simulink model "mpm_blocks"  (R2023a)
settings: Solver=VariableStepAuto  StartTime=0.0  StopTime=10.0  RelTol=1e-3
undefined symbols (not defined in the file or in its folder): conv, es
(part 1 of 3)
settings Model: Creator=bartonsa  LastModifiedBy=smbar

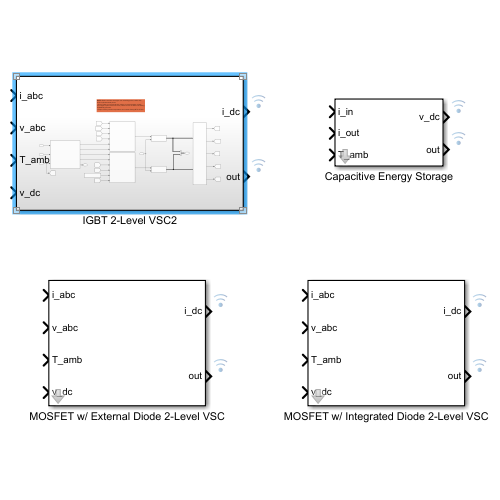
[thumbnail: Simulink's stored preview of the top-level diagram]
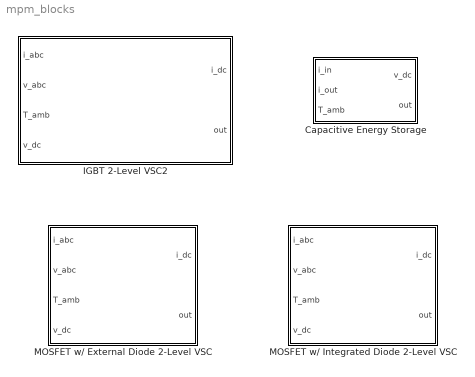
== system mpm_blocks ==
  Capacitive Energy Storage : Subsystem  mask{es=es(1)}
      mask prompts: es "Energy storage element number (i.e., es(n))"
      mask DialogControl DescGroupVar Prompt: Capacitive Energy Storage
      mask DialogControl DescTextVar Prompt: Models the thermal response of a capacitive energy storage element (i.e., supercapacitor, ultracapacitor, etc.).
  IGBT 2-Level VSC2 : Subsystem
  MOSFET w/ External Diode 2-Level VSC : Subsystem  mask{conv=conv(1)}
      mask prompts: conv "Converter name (i.e., conv(n))"
      mask DialogControl DescGroupVar Prompt: 2L VSC - MOSFET w/ ExternalDiode
      mask DialogControl DescTextVar Prompt: Models the thermal response of all switching devices in the power electronic converter.
      mask DialogControl DescTextVar2 Prompt: "out" is the junction temperature measurements for all converter devices.
      mask DialogControl DescTextVar3 Prompt: NOTE: i) Phase current is defined as flowing TOWARDS load ii) DC bus current is defined as flowing TOWARDS DC link iii) Assuming external anti-parallel diode, therefore no use of the body diode of the MOSFET.
  MOSFET w/ Integrated Diode 2-Level VSC : Subsystem  mask{conv=conv(1)}
      mask prompts: conv "Converter element (i.e., conv(n))"
      mask DialogControl DescGroupVar Prompt: 2L VSC - MOSFET w/ Integrated Diode
      mask DialogControl DescTextVar Prompt: Models the thermal response of all switching devices in the power electronic converter.
      mask DialogControl DescTextVar2 Prompt: "out" is the junction temperature measurements for all converter devices.
      mask DialogControl DescTextVar1 Prompt: NOTE: i) Phase current is defined as flowing TOWARDS load ii) DC bus current is defined as flowing TOWARDS DC link iii) Assuming no external anti-parallel diode, only the body diode of the MOSFET.

== system mpm_blocks/Capacitive Energy Storage ==
  note: Two-branch model of supercapacitor
      | Model derived from the work presented in Faranda et al., "A new parameter identification procedure for simplified double layer capacitor two-branch model," 2010
  i_in : Inport
  i_out : Inport  Port=2
  T_amb : Inport  Port=3
  Bus Creator : BusCreator  Inputs=1
  Constant : Constant  Value=es.c_0
  Constant5 : Constant  Value=es.k_v
  Constant6 : Constant  Value=es.c_2
  Divide : Product  Inputs=*/
  Divide1 : Product  Inputs=*/
  Gain : Gain  Gain=1/es.r_0
  Gain1 : Gain  Gain=1/es.r_2
  Gain2 : Gain  Gain=1/es.r_0
  Gain3 : Gain  Gain=1/es.r_2
  Gain4 : Gain  Gain=1/((1/es.r_0)+(1/es.r_2))
  Gain5 : Gain  Gain=1/es.n_p
  Gain6 : Gain  Gain=es.n_s
  Gain7 : Gain  Gain=es.r_0
  Gain8 : Gain  Gain=es.r_2
  Gain9 : Gain  Gain=es.theta
  Integrator : Integrator  InitialCondition=es.v_0
  Integrator1 : Integrator  InitialCondition=es.v_0
  Product : Product
  Square : Math  Operator=square
  Square1 : Math  Operator=square
  Sum : Sum
  Sum1 : Sum
  Sum2 : Sum  Inputs=+-
  Sum3 : Sum  Inputs=+-
  Sum4 : Sum  Inputs=+++
  Sum5 : Sum  Inputs=|++
  Sum6 : Sum
  v_dc : Outport
  out : Outport  Port=2
  wires:
  Bus Creator/1 -> out/1
  Sum5/1 -> Bus Creator/1  "T"
  T_amb/1 -> Sum5/2
  Gain9/1 -> Sum5/1
  Sum6/1 -> Gain9/1  "P_loss"
  Gain7/1 -> Sum6/1
  Gain8/1 -> Sum6/2
  [i_2] -> Square1/1
  Square1/1 -> Gain8/1
  Square/1 -> Gain7/1
  [i_1] -> Square/1
  Gain6/1 -> v_dc/1  "v_dc"
  Gain5/1 -> Sum4/1  "i_cell"
  Sum4/1 -> Gain4/1
  Gain3/1 -> Sum4/2
  Gain2/1 -> Sum4/3
  Integrator1/1 -> Gain3/1, Sum3/2  "v_2"
  Constant6/1 -> Divide1/2
  Divide1/1 -> Integrator1/1  "d_v2"
  Gain1/1 -> [i_2], Divide1/1  "i_2"
  Sum3/1 -> Gain1/1
  Integrator/1 -> Product/1, Sum2/2, Gain2/1  "v_1"
  Divide/1 -> Integrator/1  "d_v1"
  Gain/1 -> Divide/1, [i_1]  "i_1"
  Sum2/1 -> Gain/1
  Gain4/1 -> Sum3/1, Sum2/1, Gain6/1  "v_cell"
  Sum1/1 -> Divide/2
  Product/1 -> Sum1/2
  Constant5/1 -> Product/2
  Constant/1 -> Sum1/1
  i_in/1 -> Sum/1
  Sum/1 -> Gain5/1  "i_c"
  i_out/1 -> Sum/2

== system mpm_blocks/IGBT 2-Level VSC2 ==
  note: NOTE: Model considers averages over switching period, rather than electrical fundamental period.
      | - Inputs: Phase current and phase voltage (or desired phase voltage from output of pwm reference block). Phase current is defined as flowing TOWARDS generator.
      | - Output: Device junction temperature and current flowing INTO DC link.
  i_abc : Inport
  v_abc : Inport  Port=2
  T_amb : Inport  Port=3
  v_dc : Inport  Port=4
  Bus Creator : BusCreator  Inputs=2
  Constant5 : Constant  Value=conv.dev(2).Q_rr*conv.v_dc
  DIODE Loss Modeling : Subsystem
  Duty & Current Calculation : Subsystem
  IGBT Loss Modeling : Subsystem
  Thermal Impacts : Subsystem
  Thermal Model : Subsystem  mask{dev=conv.dev(1)}
      mask prompts: dev "Device number (i.e., dev(n))"
      mask DialogControl DescGroupVar Prompt: Device Thermal Model
      mask DialogControl DescTextVar Prompt: Thermal model of the specific device (assuming no thermal dependence between the switching device and diode). Note that dev(1) is typically the switch (e.g., MOSFET or IGBT) and dev(2) is the diode.
  Thermal Model1 : Subsystem  mask{dev=conv.dev(1)}
      mask prompts: dev "Device number (i.e., dev(n))"
      mask DialogControl DescGroupVar Prompt: Device Thermal Model
      mask DialogControl DescTextVar Prompt: Thermal model of the specific device (assuming no thermal dependence between the switching device and diode). Note that dev(1) is typically the switch (e.g., MOSFET or IGBT) and dev(2) is the diode.
  i_dc : Outport
  out : Outport  Port=2
  wires:
  Thermal Impacts/3(v_ce) -> [v_ce0]  "v_ce0"
  Thermal Impacts/4(r_dio) -> [r_dio]  "r_dio"
  Thermal Impacts/2(E_Qsw) -> [E_Qsw]  "E_Qsw"
  Thermal Model/1(T_j) -> Thermal Impacts/1(T_Q), Bus Creator/1  "T_Q"
  T_amb/1 -> Thermal Model/2(T_amb), Thermal Model1/2(T_amb)
  IGBT Loss Modeling/1(P_Q) -> Thermal Model/1(P_loss)  "P_M"
  Thermal Impacts/1(r_on) -> [r_on]  "r_on"
  Thermal Model1/1(T_j) -> Thermal Impacts/2(T_D), Bus Creator/2  "T_D"
  Thermal Impacts/5(v_th) -> [v_th]  "v_th"
  Bus Creator/1 -> out/1
  DIODE Loss Modeling/1(P_D) -> Thermal Model1/1(P_loss)  "P_D"
  [v_ce0] -> IGBT Loss Modeling/4(v_ce0)  "r_ds"
  [r_on] -> IGBT Loss Modeling/3(r_on)  "r_ds"
  [E_Qsw] -> IGBT Loss Modeling/2(E_sw)  "E_sw"
  [v_dc] -> IGBT Loss Modeling/1(v_dc)
  [v_dc] -> DIODE Loss Modeling/6(v_dc)  "v_dc"
  [v_th] -> DIODE Loss Modeling/4(v_th)  "v_th"
  [r_dio] -> DIODE Loss Modeling/3(r_dio)  "r_dio"
  Constant5/1 -> DIODE Loss Modeling/5(E_rr)  "E_rr"
  Duty & Current Calculation/4(i_D) -> DIODE Loss Modeling/2(i_D)  "i_D"
  Duty & Current Calculation/3(d_D) -> DIODE Loss Modeling/1(d_D)  "d_D"
  Duty & Current Calculation/2(i_Q) -> IGBT Loss Modeling/6(i_Q)  "i_Q"
  Duty & Current Calculation/1(d_Q) -> IGBT Loss Modeling/5(d_Q)  "d_Q"
  v_dc/1 -> Duty & Current Calculation/3(v_dc), [v_dc]
  i_abc/1 -> Duty & Current Calculation/1(i_s)
  v_abc/1 -> Duty & Current Calculation/2(v_s)
  Duty & Current Calculation/5(i_dc) -> i_dc/1

== system mpm_blocks/MOSFET w// External Diode 2-Level VSC ==
  note: NOTE: Model considers averages over switching period, rather than electrical fundamental period.
      | - Inputs: Phase current and phase voltage (or desired phase voltage from output of pwm reference block). Phase current is defined as flowing TOWARDS generator.
      | - Output: Device junction temperature and current flowing INTO DC link.
  i_abc : Inport
  v_abc : Inport  Port=2
  T_amb : Inport  Port=3
  v_dc : Inport  Port=4
  Bus Creator : BusCreator  Inputs=2
  Calculate Duty & Currents : Subsystem
      settings: PortSchema="{\"entries\":[{\"content\":{\"sides\":[{\"content\":{\"connectorIds\":[\"In1\",\"In2\",\"In3\"]},\"type\":\"ConnectorPlacement.EquallySpacedRectSide\",\"uuid\":\"d0795c63-5d1f-4e94-8f4f-403311821ded\"},{\"content\":{\"connectorIds\":[\"Out1\",\"Out2\",\"Out3\",\"Out4\",\"Out5\"],\"side\":\"RIGHT\"},\"type\":\"ConnectorPlacement.EquallySpacedRectSide\",\"uuid\":\"545dd18c-9caf-4cea-89fb-dae66879e352\"},{\"content\":{\"connectorIds\":[\"In4\",\"In5\",\"In6\"],\"side\":\"TOP\"},\"type\":\"ConnectorPlacement.EquallySpacedRectSide\",\"uuid\":\"9e7296e6-8783-47bd-a40b-6e0da827b704\"}]},\"type\":\"ConnectorPlacement.EquallySpacedConnector\",\"uuid\":\"8ebf9a6f-bb7f-485d-8612-a50ce46f0952\"}],\"packageUris\":[\"http://schema.mathworks.com/mf0/Connector/R2020b\"],\"version\":\"1.0\"}"
  Constant5 : Constant  Value=conv.dev(2).Q_rr*conv.v_dc
  DIODE Loss Modeling : Subsystem
  MOSFET Loss Modeling : Subsystem
  Thermal Impacts : Subsystem
  Thermal Model : Subsystem  mask{dev=conv.dev(1)}
      mask prompts: dev "Device number (i.e., dev(n))"
      mask DialogControl DescGroupVar Prompt: Device Thermal Model
      mask DialogControl DescTextVar Prompt: Thermal model of the specific device (assuming no thermal dependence between MOSFET and diode). Note that dev(1) is typically the switch (e.g., MOSFET or IGBT) and dev(2) is the diode.
  Thermal Model 1 : Subsystem  mask{dev=conv.dev(2)}
      mask prompts: dev "Device number (i.e., dev(n))"
      mask DialogControl DescGroupVar Prompt: Device Thermal Model
      mask DialogControl DescTextVar Prompt: Thermal model of the specific device (assuming no thermal dependence between MOSFET and diode). Note that dev(1) is typically the switch (e.g., MOSFET or IGBT) and dev(2) is the diode.
  i_dc : Outport
  out : Outport  Port=2
  wires:
  [r_ds] -> MOSFET Loss Modeling/3(r_ds)  "r_ds"
  DIODE Loss Modeling/1(P_D) -> Thermal Model 1/1(P_loss)  "P_D"
  T_amb/1 -> Thermal Model/2(T_amb), Thermal Model 1/2(T_amb)
  Thermal Impacts/4(v_th) -> [v_th]  "v_th"
  MOSFET Loss Modeling/1(P_M) -> Thermal Model/1(P_loss)  "P_M"
  Thermal Model/1(T_j) -> Bus Creator/1, Thermal Impacts/1(T_m)  "T_m"
  Thermal Impacts/3(r_dio) -> [r_dio]  "r_dio"
  Thermal Impacts/2(E_Qsw) -> [E_Qsw]  "E_Qsw"
  Constant5/1 -> DIODE Loss Modeling/5(E_rr)  "E_rr"
  [E_Qsw] -> MOSFET Loss Modeling/2(E_sw)  "E_sw"
  [v_th] -> DIODE Loss Modeling/4(v_th)  "v_th"
  [r_dio] -> DIODE Loss Modeling/3(r_dio)  "r_dio"
  Thermal Impacts/1(r_dson) -> [r_ds]  "r_dson"
  Calculate Duty & Currents/4(i_D) -> DIODE Loss Modeling/2(i_D)  "i_D"
  Calculate Duty & Currents/2(i_M) -> MOSFET Loss Modeling/5(i_M)  "i_M"
  Calculate Duty & Currents/1(d_M) -> MOSFET Loss Modeling/4(d_M)  "d_M"
  [r_ds] -> Calculate Duty & Currents/1(r_ds)  "r_ds"
  [v_th] -> Calculate Duty & Currents/2(v_th)  "v_th"
  [r_dio] -> Calculate Duty & Currents/3(r_dio)  "r_dio"
  Calculate Duty & Currents/3(d_D) -> DIODE Loss Modeling/1(d_D)  "d_D"
  Thermal Model 1/1(T_j) -> Thermal Impacts/2(T_d), Bus Creator/2  "T_d"
  Bus Creator/1 -> out/1
  v_dc/1 -> [v_dc], Calculate Duty & Currents/6(v_dc)
  i_abc/1 -> Calculate Duty & Currents/5(i_s)
  v_abc/1 -> Calculate Duty & Currents/4(v_s)
  Calculate Duty & Currents/5(i_dc) -> i_dc/1
  [v_dc] -> DIODE Loss Modeling/6(v_dc)  "v_dc"
  [v_dc] -> MOSFET Loss Modeling/1(v_dc)

== system mpm_blocks/MOSFET w// Integrated Diode 2-Level VSC ==
  note: NOTE: Model considers averages over switching period, rather than electrical fundamental period.
      | - Inputs: Phase current and phase voltage (or desired phase voltage from output of pwm reference block). Phase current is defined as flowing TOWARDS generator.
      | - Output: Device junction temperature and current flowing INTO DC link.
  i_abc : Inport
  v_abc : Inport  Port=2
  T_amb : Inport  Port=3
  v_dc : Inport  Port=4
  Calculate Duty & Currents : Subsystem
      settings: PortSchema="{\"entries\":[{\"content\":{\"sides\":[{\"content\":{\"connectorIds\":[\"In1\",\"In2\",\"In3\"]},\"type\":\"ConnectorPlacement.EquallySpacedRectSide\",\"uuid\":\"d0795c63-5d1f-4e94-8f4f-403311821ded\"},{\"content\":{\"connectorIds\":[\"Out1\",\"Out2\",\"Out3\",\"Out4\",\"Out5\"],\"side\":\"RIGHT\"},\"type\":\"ConnectorPlacement.EquallySpacedRectSide\",\"uuid\":\"545dd18c-9caf-4cea-89fb-dae66879e352\"},{\"content\":{\"connectorIds\":[\"In4\",\"In5\",\"In6\"],\"side\":\"TOP\"},\"type\":\"ConnectorPlacement.EquallySpacedRectSide\",\"uuid\":\"9e7296e6-8783-47bd-a40b-6e0da827b704\"}]},\"type\":\"ConnectorPlacement.EquallySpacedConnector\",\"uuid\":\"8ebf9a6f-bb7f-485d-8612-a50ce46f0952\"}],\"packageUris\":[\"http://schema.mathworks.com/mf0/Connector/R2020b\"],\"version\":\"1.0\"}"
  Constant5 : Constant  Value=conv.dev(2).Q_rr*conv.v_dc
  DE Loss Modeling : Subsystem
      settings: PortSchema="{\"entries\":[{\"content\":{\"sides\":[{\"content\":{\"connectorIds\":[\"In1\",\"In2\"]},\"type\":\"ConnectorPlacement.EquallySpacedRectSide\",\"uuid\":\"33e83bff-44ec-4dc6-9bbd-b270e5176242\"},{\"content\":{\"connectorIds\":[\"Out1\"],\"side\":\"RIGHT\"},\"type\":\"ConnectorPlacement.EquallySpacedRectSide\",\"uuid\":\"aed5fe4c-6bb6-427c-a555-2403a405bda4\"},{\"content\":{\"side\":\"TOP\"},\"type\":\"ConnectorPlacement.EquallySpacedRectSide\",\"uuid\":\"31452d4f-f1d8-4db9-9193-98611747bca7\"},{\"content\":{\"connectorIds\":[\"In3\",\"In4\",\"In5\",\"In6\"],\"side\":\"BOTTOM\"},\"type\":\"ConnectorPlacement.EquallySpacedRectSide\",\"uuid\":\"6203e927-6eb2-4c43-a609-9ad9799e7e1f\"}]},\"type\":\"ConnectorPlacement.EquallySpacedConnector\",\"uuid\":\"1e03b39d-f61e-43a7-b650-f6897d256e67\"}],\"packageUris\":[\"http://schema.mathworks.com/mf0/Connector/R2020b\"],\"version\":\"1.0\"}"
  MOSFET Loss Modeling : Subsystem
      settings: PortSchema="{\"entries\":[{\"content\":{\"sides\":[{\"content\":{\"connectorIds\":[\"In1\",\"In2\"]},\"type\":\"ConnectorPlacement.EquallySpacedRectSide\",\"uuid\":\"be72776b-5d84-4e7d-87ca-7034f165601e\"},{\"content\":{\"connectorIds\":[\"Out1\"],\"side\":\"RIGHT\"},\"type\":\"ConnectorPlacement.EquallySpacedRectSide\",\"uuid\":\"5d971d04-5834-4819-98b1-31b200ab7220\"},{\"content\":{\"connectorIds\":[\"In3\",\"In4\",\"In5\"],\"side\":\"TOP\"},\"type\":\"ConnectorPlacement.EquallySpacedRectSide\",\"uuid\":\"65eaa64d-9a38-435b-9775-bcfd5a35040a\"}]},\"type\":\"ConnectorPlacement.EquallySpacedConnector\",\"uuid\":\"b4736152-0e1c-4fdb-a43a-e03615dd6111\"}],\"packageUris\":[\"http://schema.mathworks.com/mf0/Connector/R2020b\"],\"version\":\"1.0\"}"
  Sum1 : Sum
  Thermal Impacts : Subsystem
  Thermal Model : Subsystem
  i_dc : Outport
  out : Outport  Port=2
  wires:
  MOSFET Loss Modeling/1(P_M) -> Sum1/1  "P_M"
  [r_ds] -> MOSFET Loss Modeling/3(r_ds)  "r_ds"
  DE Loss Modeling/1(P_D) -> Sum1/2  "P_D"
  T_amb/1 -> Thermal Model/2(T_amb)
  Thermal Impacts/4(v_th) -> [v_th]  "v_th"
  Sum1/1 -> Thermal Model/1(P_loss)  "P_dev"
  Thermal Model/1(T_j) -> out/1, Thermal Impacts/1(T_j)  "T_j"
  Thermal Impacts/3(r_dio) -> [r_dio]  "r_dio"
  Thermal Impacts/2(E_Qsw) -> [E_Qsw]  "E_Qsw"
  Constant5/1 -> DE Loss Modeling/6(E_rr)  "E_rr"
  [E_Qsw] -> MOSFET Loss Modeling/4(E_sw)  "E_sw"
  [v_th] -> DE Loss Modeling/4(v_th)  "v_th"
  i_abc/1 -> Calculate Duty & Currents/5(i_s)
  [r_dio] -> DE Loss Modeling/3(r_dio)  "r_dio"
  Thermal Impacts/1(r_dson) -> [r_ds]  "r_dson"
  Calculate Duty & Currents/4(i_D) -> DE Loss Modeling/2(i_D)  "i_D"
  Calculate Duty & Currents/2(i_M) -> MOSFET Loss Modeling/2(i_M)  "i_M"
  Calculate Duty & Currents/1(d_M) -> MOSFET Loss Modeling/1(d_M)  "d_M"
  v_abc/1 -> Calculate Duty & Currents/4(v_s)
  [r_ds] -> Calculate Duty & Currents/1(r_ds)  "r_ds"
  [v_th] -> Calculate Duty & Currents/2(v_th)  "v_th"
  [r_dio] -> Calculate Duty & Currents/3(r_dio)  "r_dio"
  Calculate Duty & Currents/3(d_D) -> DE Loss Modeling/1(d_D)  "d_D"
  v_dc/1 -> [v_dc], Calculate Duty & Currents/6(v_dc)
  Calculate Duty & Currents/5(i_dc) -> i_dc/1
  [v_dc] -> MOSFET Loss Modeling/5(v_dc)  "v_dc"
  [v_dc] -> DE Loss Modeling/5(v_dc)  "v_dc"

== system mpm_blocks/IGBT 2-Level VSC2/DIODE Loss Modeling ==
  d_D : Inport
  i_D : Inport  Port=2
  r_dio : Inport  Port=3
  v_th : Inport  Port=4
  E_rr : Inport  Port=5
  v_dc : Inport  Port=6
  Gain : Gain  Gain=1/conv.dev(2).V_ref
  Gain3 : Gain  Gain=1/conv.dev(2).I_ref
  Gain4 : Gain  Gain=conv.f_sw
  Product : Product
  Product3 : Product  Inputs=3
  Product6 : Product  Inputs=3
  Product8 : Product
  Sqrt : Sqrt
  Square2 : Math  Operator=square
  Sum : Sum
  Sum2 : Sum
  P_D : Outport
  wires:
  v_dc/1 -> Gain/1
  Product/1 -> Gain3/1, Product8/1  "i_D_avg"
  i_D/1 -> Square2/1, Product/2  "i_D"
  d_D/1 -> Product6/2, Product/1  "d_D"
  Sqrt/1 -> Product3/3  "iscale"
  Gain3/1 -> Sqrt/1
  Gain/1 -> Product3/2  "vscale"
  Product6/1 -> Sum/1
  Product8/1 -> Sum/2
  Square2/1 -> Product6/3
  Sum/1 -> Sum2/1  "P_CD"
  Gain4/1 -> Sum2/2  "P_SD"
  r_dio/1 -> Product6/1
  Product3/1 -> Gain4/1
  Sum2/1 -> P_D/1  "P_D"
  v_th/1 -> Product8/2
  E_rr/1 -> Product3/1

== system mpm_blocks/IGBT 2-Level VSC2/Duty & Current Calculation ==
  note: Duty Cycle Estimation
  i_s : Inport
  v_s : Inport  Port=2
  v_dc : Inport  Port=3
  Calculate Device Currents : MATLAB Function  TreatAsAtomicUnit=on
  Constant : Constant
  Constant2 : Constant
  Constant3 : Constant  Value=2*conv.t_d*conv.f_sw
  Constant4 : Constant  Value=2*conv.t_d*conv.f_sw
  Divide : Product  Inputs=*/
  Gain : Gain  Gain=-1
  Gain1 : Gain  Gain=1/2
  Gain2 : Gain  Gain=2
  MATLAB Function3 : MATLAB Function  TreatAsAtomicUnit=on
  Mux : Mux  Inputs=2
  Product : Product
  Product1 : Product
  Selector : Selector  InputPortWidth=6  IndexOptions=Index vector (dialog)  Indices=[1 2 3]  OutputSizes=1
  Selector1 : Selector  InputPortWidth=6  IndexOptions=Index vector (dialog)  Indices=[1 2 3]  OutputSizes=1
  Subtract : Sum  Inputs=+-
  Subtract1 : Sum  Inputs=-+-
  Sum of Elements : Sum  Inputs=+
  Sum1 : Sum  Inputs=+-+
  d_Q : Outport
  i_Q : Outport  Port=2
  d_D : Outport  Port=3
  i_D : Outport  Port=4
  i_dc : Outport  Port=5
  wires:
  Calculate Device Currents/4(d_D) -> d_D/1, Product1/2  "d_D"
  Calculate Device Currents/3(i_D) -> Product1/1, i_D/1  "i_D"
  Calculate Device Currents/1(i_Q) -> Product/1, i_Q/1  "i_Q"
  Selector1/1 -> Subtract/2
  Selector/1 -> Subtract/1
  Subtract/1 -> Sum of Elements/1  "diff"
  Sum of Elements/1 -> Gain/1
  Gain/1 -> i_dc/1  "i_dc"
  Product/1 -> Selector/1  "iQ_avg"
  Product1/1 -> Selector1/1  "iD_avg"
  i_s/1 -> Calculate Device Currents/3(i_s)
  Mux/1 -> Calculate Device Currents/1(d_Q)  "d_Q"
  Calculate Device Currents/2(d_Qnew) -> d_Q/1, Product/2  "d_Q"
  MATLAB Function3/1(y) -> Sum1/3
  Constant/1 -> Sum1/1
  v_s/1 -> Gain2/1  "v_s"
  Constant2/1 -> Subtract1/2
  Gain1/1 -> Mux/1, Subtract1/1  "d_H"
  Divide/1 -> MATLAB Function3/1(u)  "m_a"
  Sum1/1 -> Gain1/1
  Constant4/1 -> Calculate Device Currents/2(d_deadTime), Subtract1/3  "d_deadTime"
  Subtract1/1 -> Mux/2  "d_L"
  Constant3/1 -> Sum1/2
  Gain2/1 -> Divide/1
  v_dc/1 -> Divide/2

== system mpm_blocks/IGBT 2-Level VSC2/IGBT Loss Modeling ==
  note: P_cond = v_ce*I_avg + r_on*I_rms^2
  v_dc : Inport
  E_sw : Inport  Port=2
  r_on : Inport  Port=3
  v_ce0 : Inport  Port=4
  d_Q : Inport  Port=5
  i_Q : Inport  Port=6
  Abs : Abs  SaturateOnIntegerOverflow=off
  Constant : Constant  Value=conv.dev(1).k_v
  Gain : Gain  Gain=1/conv.dev(1).V_ref
  Gain1 : Gain  Gain=conv.f_sw
  Gain2 : Gain  Gain=1/conv.dev(1).I_ref
  Power : Math  Operator=pow
  Product : Product
  Product1 : Product
  Product10 : Product  Inputs=3
  Product2 : Product
  Product4 : Product  Inputs=3
  Square : Math  Operator=square
  Sum : Sum
  Sum1 : Sum
  P_Q : Outport
  wires:
  Product1/1 -> Sum/1
  Product4/1 -> Sum/2  "P_CQ"
  Product2/1 -> Product1/2  "i_Qavg"
  v_ce0/1 -> Product1/1
  v_dc/1 -> Gain/1
  Gain/1 -> Power/1
  Constant/1 -> Power/2
  Product/1 -> Abs/1  "i_Qavg"
  d_Q/1 -> Product2/1, Product4/2, Product/2  "d"
  Abs/1 -> Gain2/1
  Sum1/1 -> P_Q/1  "P_Q"
  E_sw/1 -> Product10/1
  i_Q/1 -> Product/1, Square/1, Product2/2  "i_Q"
  Gain1/1 -> Sum1/2  "P_SQ"
  r_on/1 -> Product4/1
  Power/1 -> Product10/3  "vscale"
  Product10/1 -> Gain1/1
  Square/1 -> Product4/3
  Gain2/1 -> Product10/2  "iscale"
  Sum/1 -> Sum1/1  "P_CQ"

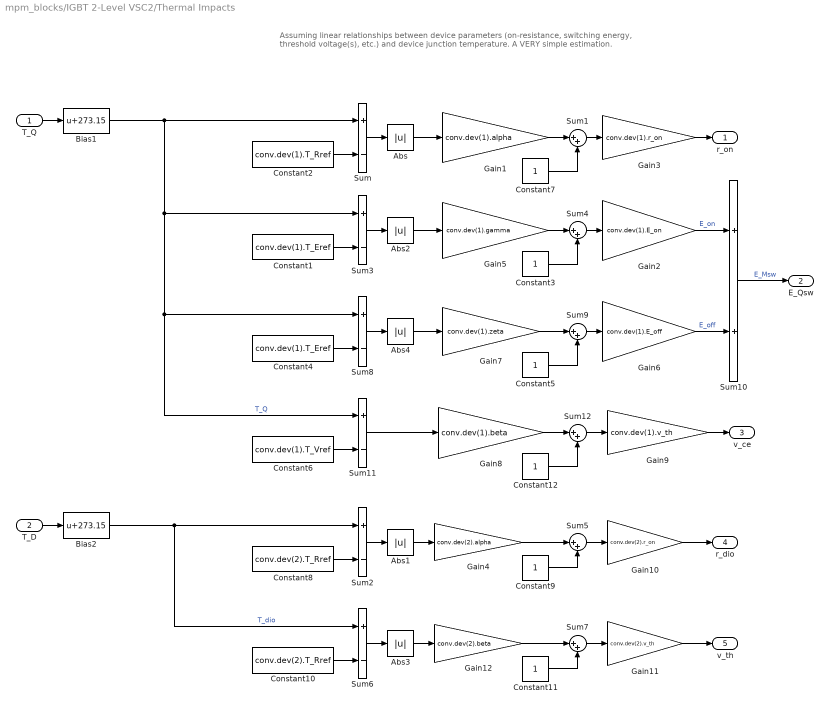
== system mpm_blocks/IGBT 2-Level VSC2/Thermal Impacts ==
  note: Assuming linear relationships between device parameters (on-resistance, switching energy, threshold voltage(s), etc.) and device junction temperature. A VERY simple estimation.
  T_Q : Inport
  T_D : Inport  Port=2
  Abs{,1..4} (5 alike) : Abs  SaturateOnIntegerOverflow=off
  Bias1 : Bias  Bias=273.15  SaturateOnIntegerOverflow=off
  Bias2 : Bias  Bias=273.15  SaturateOnIntegerOverflow=off
  Constant1 : Constant  Value=conv.dev(1).T_Eref
  Constant10 : Constant  Value=conv.dev(2).T_Rref
  Constant{3,5,7,9,11..12} (6 alike) : Constant
  Constant2 : Constant  Value=conv.dev(1).T_Rref
  Constant4 : Constant  Value=conv.dev(1).T_Eref
  Constant6 : Constant  Value=conv.dev(1).T_Vref
  Constant8 : Constant  Value=conv.dev(2).T_Rref
  Gain1 : Gain  Gain=conv.dev(1).alpha
  Gain10 : Gain  Gain=conv.dev(2).r_on
  Gain11 : Gain  Gain=conv.dev(2).v_th
  Gain12 : Gain  Gain=conv.dev(2).beta
  Gain2 : Gain  Gain=conv.dev(1).E_on
  Gain3 : Gain  Gain=conv.dev(1).r_on
  Gain4 : Gain  Gain=conv.dev(2).alpha
  Gain5 : Gain  Gain=conv.dev(1).gamma
  Gain6 : Gain  Gain=conv.dev(1).E_off
  Gain7 : Gain  Gain=conv.dev(1).zeta
  Gain8 : Gain  Gain=conv.dev(1).beta
  Gain9 : Gain  Gain=conv.dev(1).v_th
  Sum{,2..3,6,8,11} (6 alike) : Sum  Inputs=+-
  Sum{1,4..5,7,9,12} (6 alike) : Sum  Inputs=|++
  Sum10 : Sum
  r_on : Outport
  E_Qsw : Outport  Port=2
  v_ce : Outport  Port=3
  r_dio : Outport  Port=4
  v_th : Outport  Port=5
  wires:
  Sum11/1 -> Gain8/1
  Constant12/1 -> Sum12/2
  Sum12/1 -> Gain9/1
  Gain9/1 -> v_ce/1
  Gain8/1 -> Sum12/1
  Constant6/1 -> Sum11/2
  T_D/1 -> Bias2/1
  Bias2/1 -> Sum2/1, Sum6/1  "T_dio"
  T_Q/1 -> Bias1/1
  Bias1/1 -> Sum/1, Sum3/1, Sum8/1, Sum11/1  "T_Q"
  Sum10/1 -> E_Qsw/1  "E_Msw"
  Gain7/1 -> Sum9/1
  Sum8/1 -> Abs4/1
  Constant5/1 -> Sum9/2
  Sum9/1 -> Gain6/1
  Gain6/1 -> Sum10/2  "E_off"
  Abs4/1 -> Gain7/1
  Constant4/1 -> Sum8/2
  Constant1/1 -> Sum3/2
  Sum4/1 -> Gain2/1
  Gain2/1 -> Sum10/1  "E_on"
  Abs2/1 -> Gain5/1
  Gain5/1 -> Sum4/1
  Constant3/1 -> Sum4/2
  Sum3/1 -> Abs2/1
  Abs3/1 -> Gain12/1
  Constant2/1 -> Sum/2
  Constant11/1 -> Sum7/2
  Gain11/1 -> v_th/1
  Sum7/1 -> Gain11/1
  Constant10/1 -> Sum6/2
  Gain12/1 -> Sum7/1
  Sum6/1 -> Abs3/1
  Abs/1 -> Gain1/1
  Gain1/1 -> Sum1/1
  Sum1/1 -> Gain3/1
  Constant7/1 -> Sum1/2
  Sum2/1 -> Abs1/1
  Constant8/1 -> Sum2/2
  Constant9/1 -> Sum5/2
  Gain4/1 -> Sum5/1
  Abs1/1 -> Gain4/1
  Sum5/1 -> Gain10/1
  Gain10/1 -> r_dio/1
  Gain3/1 -> r_on/1
  Sum/1 -> Abs/1

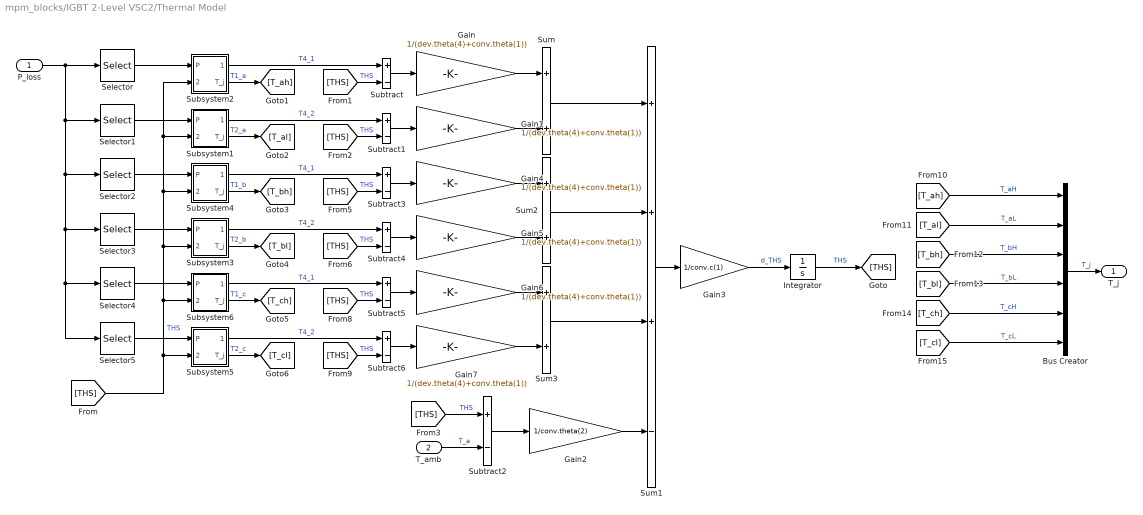
== system mpm_blocks/IGBT 2-Level VSC2/Thermal Model ==
  P_loss : Inport
  T_amb : Inport  Port=2
  Bus Creator : BusCreator  Inputs=6
  Gain{,1,4..7} (6 alike) : Gain  Gain=1/(dev.theta(4)+conv.theta(1))
  Gain2 : Gain  Gain=1/conv.theta(2)
  Gain3 : Gain  Gain=1/conv.c(1)
  Integrator : Integrator  InitialCondition=conv.T_init-273.15
  Selector : Selector  InputPortWidth=6  IndexOptions=Index vector (dialog)  Indices=1  OutputSizes=1
  Selector1 : Selector  InputPortWidth=6  IndexOptions=Index vector (dialog)  Indices=4  OutputSizes=1
  Selector2 : Selector  InputPortWidth=6  IndexOptions=Index vector (dialog)  Indices=2  OutputSizes=1
  Selector3 : Selector  InputPortWidth=6  IndexOptions=Index vector (dialog)  Indices=5  OutputSizes=1
  Selector4 : Selector  InputPortWidth=6  IndexOptions=Index vector (dialog)  Indices=3  OutputSizes=1
  Selector5 : Selector  InputPortWidth=6  IndexOptions=Index vector (dialog)  Indices=6  OutputSizes=1
  Subsystem1 : Subsystem
  Subsystem2 : Subsystem
  Subsystem3 : Subsystem
  Subsystem4 : Subsystem
  Subsystem5 : Subsystem
  Subsystem6 : Subsystem
  Subtract{,1..6} (7 alike) : Sum  Inputs=+-
  Sum : Sum
  Sum1 : Sum  Inputs=+++-
  Sum2 : Sum
  Sum3 : Sum
  T_j : Outport
  wires:
  [THS] -> Subsystem5/2(THS), Subsystem6/2(THS), Subsystem3/2(THS), Subsystem4/2(THS), Subsystem1/2(THS), Subsystem2/2(THS)  "THS"
  Selector2/1 -> Subsystem4/1(P)
  Selector1/1 -> Subsystem1/1(P)
  Selector5/1 -> Subsystem5/1(P)
  Selector4/1 -> Subsystem6/1(P)
  Selector3/1 -> Subsystem3/1(P)
  Selector/1 -> Subsystem2/1(P)
  [T_bh] -> Bus Creator/3  "T_bH"
  Bus Creator/1 -> T_j/1  "T_j"
  [T_cl] -> Bus Creator/6  "T_cL"
  [T_al] -> Bus Creator/2  "T_aL"
  [T_bl] -> Bus Creator/4  "T_bL"
  [T_ch] -> Bus Creator/5  "T_cH"
  [T_ah] -> Bus Creator/1  "T_aH"
  P_loss/1 -> Selector/1, Selector1/1, Selector2/1, Selector3/1, Selector4/1, Selector5/1
  Subsystem6/2(T_j) -> [T_ch]  "T1_c"
  Subtract1/1 -> Gain1/1
  Subtract3/1 -> Gain4/1
  Gain3/1 -> Integrator/1  "d_THS"
  Sum2/1 -> Sum1/2
  Subsystem4/1(T_c) -> Subtract3/1  "T4_1"
  Subsystem3/1(T_c) -> Subtract4/1  "T4_2"
  Sum3/1 -> Sum1/3
  Subsystem4/2(T_j) -> [T_bh]  "T1_b"
  Gain1/1 -> Sum/2
  Gain5/1 -> Sum2/2
  [THS] -> Subtract/2  "THS"
  Subtract2/1 -> Gain2/1
  [THS] -> Subtract3/2  "THS"
  Subtract5/1 -> Gain6/1
  [THS] -> Subtract4/2  "THS"
  Subsystem5/1(T_c) -> Subtract6/1  "T4_2"
  Gain4/1 -> Sum2/1
  Sum/1 -> Sum1/1
  Subsystem3/2(T_j) -> [T_bl]  "T2_b"
  Subtract4/1 -> Gain5/1
  Integrator/1 -> [THS]  "THS"
  Sum1/1 -> Gain3/1
  Gain2/1 -> Sum1/4
  T_amb/1 -> Subtract2/2  "T_a"
  [THS] -> Subtract1/2  "THS"
  Subsystem1/2(T_j) -> [T_al]  "T2_a"
  Gain/1 -> Sum/1
  Gain6/1 -> Sum3/1
  [THS] -> Subtract2/1  "THS"
  [THS] -> Subtract6/2  "THS"
  Subsystem5/2(T_j) -> [T_cl]  "T2_c"
  Subtract6/1 -> Gain7/1
  Gain7/1 -> Sum3/2
  [THS] -> Subtract5/2  "THS"
  Subsystem6/1(T_c) -> Subtract5/1  "T4_1"
  Subsystem2/2(T_j) -> [T_ah]  "T1_a"
  Subtract/1 -> Gain/1
  Subsystem1/1(T_c) -> Subtract1/1  "T4_2"
  Subsystem2/1(T_c) -> Subtract/1  "T4_1"

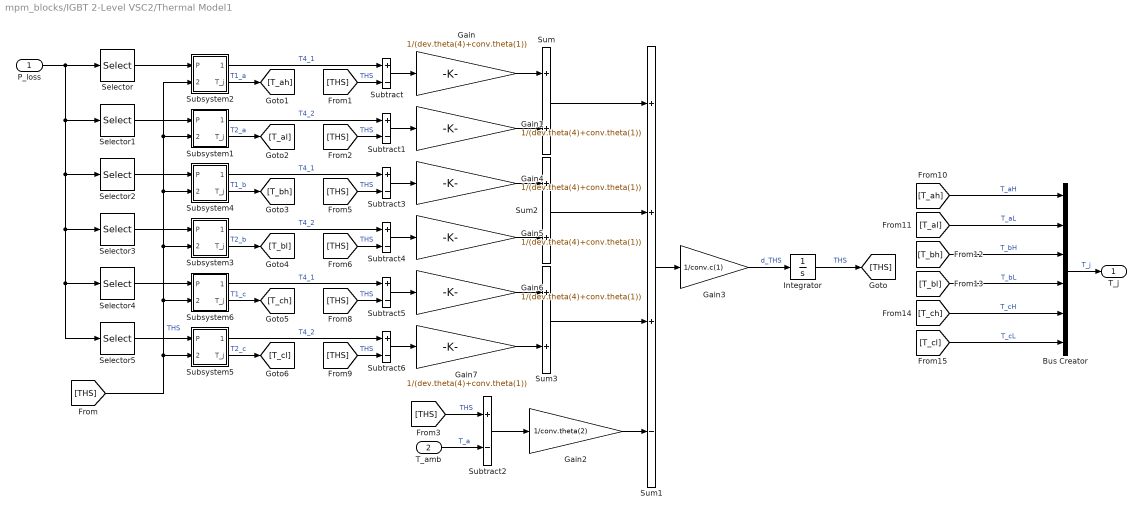
== system mpm_blocks/IGBT 2-Level VSC2/Thermal Model1 ==
  P_loss : Inport
  T_amb : Inport  Port=2
  Bus Creator : BusCreator  Inputs=6
  Gain{,1,4..7} (6 alike) : Gain  Gain=1/(dev.theta(4)+conv.theta(1))
  Gain2 : Gain  Gain=1/conv.theta(2)
  Gain3 : Gain  Gain=1/conv.c(1)
  Integrator : Integrator  InitialCondition=conv.T_init-273.15
  Selector : Selector  InputPortWidth=6  IndexOptions=Index vector (dialog)  Indices=1  OutputSizes=1
  Selector1 : Selector  InputPortWidth=6  IndexOptions=Index vector (dialog)  Indices=4  OutputSizes=1
  Selector2 : Selector  InputPortWidth=6  IndexOptions=Index vector (dialog)  Indices=2  OutputSizes=1
  Selector3 : Selector  InputPortWidth=6  IndexOptions=Index vector (dialog)  Indices=5  OutputSizes=1
  Selector4 : Selector  InputPortWidth=6  IndexOptions=Index vector (dialog)  Indices=3  OutputSizes=1
  Selector5 : Selector  InputPortWidth=6  IndexOptions=Index vector (dialog)  Indices=6  OutputSizes=1
  Subsystem1 : Subsystem
  Subsystem2 : Subsystem
  Subsystem3 : Subsystem
  Subsystem4 : Subsystem
  Subsystem5 : Subsystem
  Subsystem6 : Subsystem
  Subtract{,1..6} (7 alike) : Sum  Inputs=+-
  Sum : Sum
  Sum1 : Sum  Inputs=+++-
  Sum2 : Sum
  Sum3 : Sum
  T_j : Outport
  wires:
  Subsystem2/1(T_c) -> Subtract/1  "T4_1"
  Subsystem1/1(T_c) -> Subtract1/1  "T4_2"
  Subtract/1 -> Gain/1
  Subsystem2/2(T_j) -> [T_ah]  "T1_a"
  Subsystem6/1(T_c) -> Subtract5/1  "T4_1"
  [THS] -> Subtract5/2  "THS"
  Gain7/1 -> Sum3/2
  Subtract6/1 -> Gain7/1
  Subsystem5/2(T_j) -> [T_cl]  "T2_c"
  [THS] -> Subtract6/2  "THS"
  [THS] -> Subtract2/1  "THS"
  Gain6/1 -> Sum3/1
  Gain/1 -> Sum/1
  Subsystem1/2(T_j) -> [T_al]  "T2_a"
  [THS] -> Subtract1/2  "THS"
  T_amb/1 -> Subtract2/2  "T_a"
  Gain2/1 -> Sum1/4
  Sum1/1 -> Gain3/1
  Integrator/1 -> [THS]  "THS"
  Subtract4/1 -> Gain5/1
  Subsystem3/2(T_j) -> [T_bl]  "T2_b"
  Sum/1 -> Sum1/1
  Gain4/1 -> Sum2/1
  Subsystem5/1(T_c) -> Subtract6/1  "T4_2"
  [THS] -> Subtract4/2  "THS"
  Subtract5/1 -> Gain6/1
  [THS] -> Subtract3/2  "THS"
  Subtract2/1 -> Gain2/1
  [THS] -> Subtract/2  "THS"
  Gain5/1 -> Sum2/2
  Gain1/1 -> Sum/2
  Subsystem4/2(T_j) -> [T_bh]  "T1_b"
  Sum3/1 -> Sum1/3
  Subsystem3/1(T_c) -> Subtract4/1  "T4_2"
  Subsystem4/1(T_c) -> Subtract3/1  "T4_1"
  Sum2/1 -> Sum1/2
  Gain3/1 -> Integrator/1  "d_THS"
  Subtract3/1 -> Gain4/1
  Subtract1/1 -> Gain1/1
  Subsystem6/2(T_j) -> [T_ch]  "T1_c"
  P_loss/1 -> Selector5/1, Selector4/1, Selector3/1, Selector2/1, Selector1/1, Selector/1
  [T_ah] -> Bus Creator/1  "T_aH"
  [T_ch] -> Bus Creator/5  "T_cH"
  [T_bl] -> Bus Creator/4  "T_bL"
  [T_al] -> Bus Creator/2  "T_aL"
  [T_cl] -> Bus Creator/6  "T_cL"
  Bus Creator/1 -> T_j/1  "T_j"
  [T_bh] -> Bus Creator/3  "T_bH"
  Selector/1 -> Subsystem2/1(P)
  Selector3/1 -> Subsystem3/1(P)
  Selector4/1 -> Subsystem6/1(P)
  Selector5/1 -> Subsystem5/1(P)
  Selector1/1 -> Subsystem1/1(P)
  Selector2/1 -> Subsystem4/1(P)
  [THS] -> Subsystem2/2(THS), Subsystem1/2(THS), Subsystem4/2(THS), Subsystem3/2(THS), Subsystem6/2(THS), Subsystem5/2(THS)  "THS"

== system mpm_blocks/MOSFET w// External Diode 2-Level VSC/Calculate Duty & Currents ==
  r_ds : Inport
  v_th : Inport  Port=2
  r_dio : Inport  Port=3
  v_s : Inport  Port=4
  i_s : Inport  Port=5
  v_dc : Inport  Port=6
  Calculate Device Currents : MATLAB Function  TreatAsAtomicUnit=on
  Duty Cycle Estimation : Subsystem
  Gain : Gain  Gain=-1
  Product : Product
  Product1 : Product
  Selector : Selector  InputPortWidth=6  IndexOptions=Index vector (dialog)  Indices=[1 2 3]  OutputSizes=1
  Selector1 : Selector  InputPortWidth=6  IndexOptions=Index vector (dialog)  Indices=[1 2 3]  OutputSizes=1
  Subtract : Sum  Inputs=+-
  Sum of Elements : Sum  Inputs=+
  d_M : Outport
  i_M : Outport  Port=2
  d_D : Outport  Port=3
  i_D : Outport  Port=4
  i_dc : Outport  Port=5
  wires:
  r_dio/1 -> Calculate Device Currents/6(r_dio)
  v_s/1 -> Duty Cycle Estimation/2(v_s)
  Calculate Device Currents/1(i_M) -> i_M/1, Product/2  "i_M"
  Duty Cycle Estimation/2(d_deadTime) -> Calculate Device Currents/2(d_deadTime)  "d_deadTime"
  r_ds/1 -> Calculate Device Currents/4(r_ds)
  v_th/1 -> Calculate Device Currents/5(v_th)
  Duty Cycle Estimation/1(d_M) -> d_M/1, Product/1, Calculate Device Currents/1(d_M)  "d_M"
  i_s/1 -> Calculate Device Currents/3(i_s)
  v_dc/1 -> Duty Cycle Estimation/1(v_dc)
  Calculate Device Currents/3(d_D) -> Product1/2, d_D/1  "d_D"
  Calculate Device Currents/2(i_D) -> Product1/1, i_D/1  "i_D"
  Product1/1 -> Selector1/1
  Product/1 -> Selector/1
  Gain/1 -> i_dc/1  "i_dc"
  Sum of Elements/1 -> Gain/1
  Subtract/1 -> Sum of Elements/1  "diff"
  Selector/1 -> Subtract/1
  Selector1/1 -> Subtract/2

== system mpm_blocks/MOSFET w// External Diode 2-Level VSC/DIODE Loss Modeling ==
  d_D : Inport
  i_D : Inport  Port=2
  r_dio : Inport  Port=3
  v_th : Inport  Port=4
  E_rr : Inport  Port=5
  v_dc : Inport  Port=6
  Gain : Gain  Gain=1/conv.dev(2).V_ref
  Gain3 : Gain  Gain=1/conv.dev(2).I_ref
  Gain4 : Gain  Gain=conv.f_sw
  Product : Product
  Product3 : Product  Inputs=3
  Product6 : Product  Inputs=3
  Product8 : Product
  Sqrt : Sqrt
  Square2 : Math  Operator=square
  Sum : Sum
  Sum2 : Sum
  P_D : Outport
  wires:
  E_rr/1 -> Product3/1
  v_th/1 -> Product8/2
  Sum2/1 -> P_D/1  "P_D"
  Product3/1 -> Gain4/1
  r_dio/1 -> Product6/1
  Gain4/1 -> Sum2/2  "P_SD"
  Sum/1 -> Sum2/1  "P_CD"
  Square2/1 -> Product6/3
  Product8/1 -> Sum/2
  Product6/1 -> Sum/1
  Gain/1 -> Product3/2  "vscale"
  Gain3/1 -> Sqrt/1
  Sqrt/1 -> Product3/3  "iscale"
  d_D/1 -> Product/1, Product6/2  "d_D"
  i_D/1 -> Product/2, Square2/1  "i_D"
  Product/1 -> Product8/1, Gain3/1  "i_D_avg"
  v_dc/1 -> Gain/1

== system mpm_blocks/MOSFET w// External Diode 2-Level VSC/MOSFET Loss Modeling ==
  v_dc : Inport
  E_sw : Inport  Port=2
  r_ds : Inport  Port=3
  d_M : Inport  Port=4
  i_M : Inport  Port=5
  Abs : Abs  SaturateOnIntegerOverflow=off
  Constant : Constant  Value=conv.dev(1).k_v
  Gain : Gain  Gain=1/conv.dev(1).V_ref
  Gain1 : Gain  Gain=conv.f_sw
  Gain2 : Gain  Gain=1/conv.dev(1).I_ref
  Power : Math  Operator=pow
  Product : Product
  Product10 : Product  Inputs=3
  Product4 : Product  Inputs=3
  Square : Math  Operator=square
  Sum1 : Sum
  P_M : Outport
  wires:
  Product4/1 -> Sum1/1  "P_CM"
  Gain2/1 -> Product10/2  "iscale"
  Square/1 -> Product4/3
  Product10/1 -> Gain1/1
  Power/1 -> Product10/3  "vscale"
  r_ds/1 -> Product4/1
  Gain1/1 -> Sum1/2  "P_SM"
  i_M/1 -> Square/1, Product/1  "i_M"
  E_sw/1 -> Product10/1
  Sum1/1 -> P_M/1  "P_M"
  Abs/1 -> Gain2/1
  d_M/1 -> Product/2, Product4/2  "d"
  Product/1 -> Abs/1
  Constant/1 -> Power/2
  Gain/1 -> Power/1
  v_dc/1 -> Gain/1

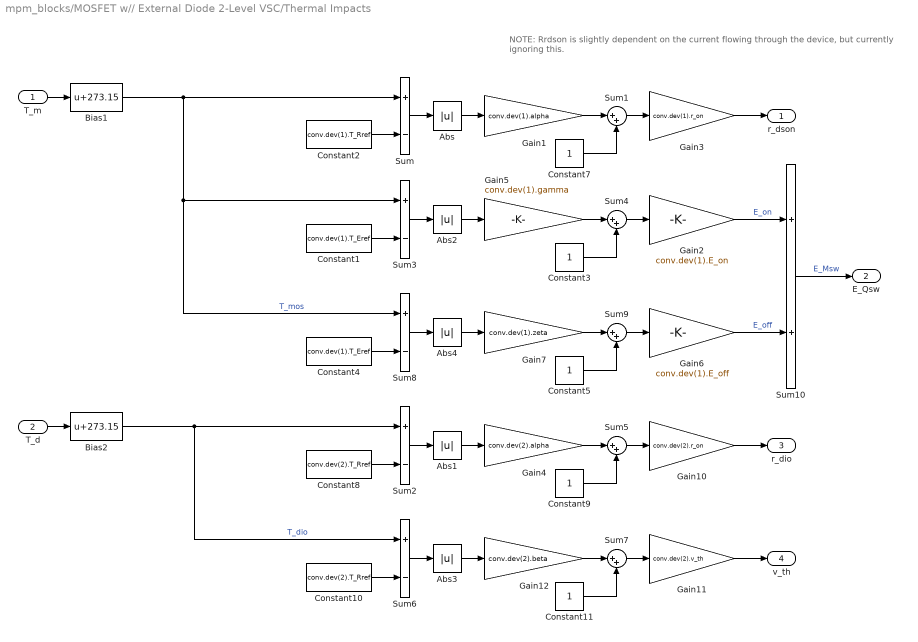
== system mpm_blocks/MOSFET w// External Diode 2-Level VSC/Thermal Impacts ==
  note: NOTE: Rrdson is slightly dependent on the current flowing through the device, but currently ignoring this.
  T_m : Inport
  T_d : Inport  Port=2
  Abs{,1..4} (5 alike) : Abs  SaturateOnIntegerOverflow=off
  Bias1 : Bias  Bias=273.15  SaturateOnIntegerOverflow=off
  Bias2 : Bias  Bias=273.15  SaturateOnIntegerOverflow=off
  Constant1 : Constant  Value=conv.dev(1).T_Eref
  Constant10 : Constant  Value=conv.dev(2).T_Rref
  Constant{3,5,7,9,11} (5 alike) : Constant
  Constant2 : Constant  Value=conv.dev(1).T_Rref
  Constant4 : Constant  Value=conv.dev(1).T_Eref
  Constant8 : Constant  Value=conv.dev(2).T_Rref
  Gain1 : Gain  Gain=conv.dev(1).alpha
  Gain10 : Gain  Gain=conv.dev(2).r_on
  Gain11 : Gain  Gain=conv.dev(2).v_th
  Gain12 : Gain  Gain=conv.dev(2).beta
  Gain2 : Gain  Gain=conv.dev(1).E_on
  Gain3 : Gain  Gain=conv.dev(1).r_on
  Gain4 : Gain  Gain=conv.dev(2).alpha
  Gain5 : Gain  Gain=conv.dev(1).gamma
  Gain6 : Gain  Gain=conv.dev(1).E_off
  Gain7 : Gain  Gain=conv.dev(1).zeta
  Sum{,2..3,6,8} (5 alike) : Sum  Inputs=+-
  Sum{1,4..5,7,9} (5 alike) : Sum  Inputs=|++
  Sum10 : Sum
  r_dson : Outport
  E_Qsw : Outport  Port=2
  r_dio : Outport  Port=3
  v_th : Outport  Port=4
  wires:
  Sum/1 -> Abs/1
  Gain3/1 -> r_dson/1
  Gain10/1 -> r_dio/1
  Sum5/1 -> Gain10/1
  Abs1/1 -> Gain4/1
  Gain4/1 -> Sum5/1
  Constant9/1 -> Sum5/2
  Constant8/1 -> Sum2/2
  Sum2/1 -> Abs1/1
  Constant7/1 -> Sum1/2
  Sum1/1 -> Gain3/1
  Gain1/1 -> Sum1/1
  Abs/1 -> Gain1/1
  Sum6/1 -> Abs3/1
  Gain12/1 -> Sum7/1
  Constant10/1 -> Sum6/2
  Sum7/1 -> Gain11/1
  Gain11/1 -> v_th/1
  Constant11/1 -> Sum7/2
  Constant2/1 -> Sum/2
  Abs3/1 -> Gain12/1
  Sum3/1 -> Abs2/1
  Constant3/1 -> Sum4/2
  Gain5/1 -> Sum4/1
  Abs2/1 -> Gain5/1
  Gain2/1 -> Sum10/1  "E_on"
  Sum4/1 -> Gain2/1
  Constant1/1 -> Sum3/2
  Constant4/1 -> Sum8/2
  Abs4/1 -> Gain7/1
  Gain6/1 -> Sum10/2  "E_off"
  Sum9/1 -> Gain6/1
  Constant5/1 -> Sum9/2
  Sum8/1 -> Abs4/1
  Gain7/1 -> Sum9/1
  Sum10/1 -> E_Qsw/1  "E_Msw"
  Bias1/1 -> Sum8/1, Sum3/1, Sum/1  "T_mos"
  T_m/1 -> Bias1/1
  Bias2/1 -> Sum6/1, Sum2/1  "T_dio"
  T_d/1 -> Bias2/1

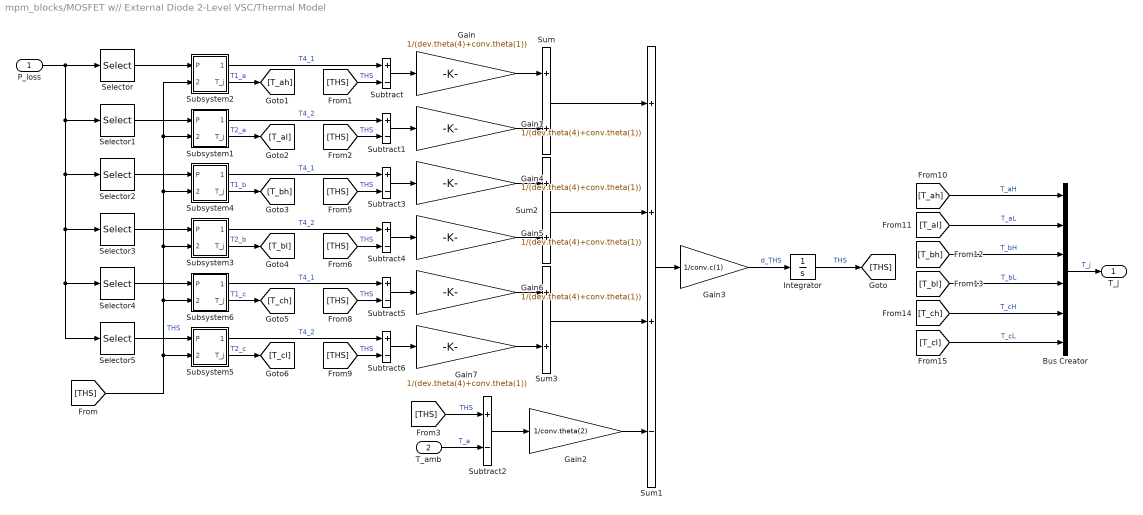
== system mpm_blocks/MOSFET w// External Diode 2-Level VSC/Thermal Model ==
  P_loss : Inport
  T_amb : Inport  Port=2
  Bus Creator : BusCreator  Inputs=6
  Gain{,1,4..7} (6 alike) : Gain  Gain=1/(dev.theta(4)+conv.theta(1))
  Gain2 : Gain  Gain=1/conv.theta(2)
  Gain3 : Gain  Gain=1/conv.c(1)
  Integrator : Integrator  InitialCondition=conv.T_init-273.15
  Selector : Selector  InputPortWidth=6  IndexOptions=Index vector (dialog)  Indices=1  OutputSizes=1
  Selector1 : Selector  InputPortWidth=6  IndexOptions=Index vector (dialog)  Indices=4  OutputSizes=1
  Selector2 : Selector  InputPortWidth=6  IndexOptions=Index vector (dialog)  Indices=2  OutputSizes=1
  Selector3 : Selector  InputPortWidth=6  IndexOptions=Index vector (dialog)  Indices=5  OutputSizes=1
  Selector4 : Selector  InputPortWidth=6  IndexOptions=Index vector (dialog)  Indices=3  OutputSizes=1
  Selector5 : Selector  InputPortWidth=6  IndexOptions=Index vector (dialog)  Indices=6  OutputSizes=1
  Subsystem1 : Subsystem
  Subsystem2 : Subsystem
  Subsystem3 : Subsystem
  Subsystem4 : Subsystem
  Subsystem5 : Subsystem
  Subsystem6 : Subsystem
  Subtract{,1..6} (7 alike) : Sum  Inputs=+-
  Sum : Sum
  Sum1 : Sum  Inputs=+++-
  Sum2 : Sum
  Sum3 : Sum
  T_j : Outport
  wires:
  Subsystem2/1(T_c) -> Subtract/1  "T4_1"
  Subsystem1/1(T_c) -> Subtract1/1  "T4_2"
  Subtract/1 -> Gain/1
  Subsystem2/2(T_j) -> [T_ah]  "T1_a"
  Subsystem6/1(T_c) -> Subtract5/1  "T4_1"
  [THS] -> Subtract5/2  "THS"
  Gain7/1 -> Sum3/2
  Subtract6/1 -> Gain7/1
  Subsystem5/2(T_j) -> [T_cl]  "T2_c"
  [THS] -> Subtract6/2  "THS"
  [THS] -> Subtract2/1  "THS"
  Gain6/1 -> Sum3/1
  Gain/1 -> Sum/1
  Subsystem1/2(T_j) -> [T_al]  "T2_a"
  [THS] -> Subtract1/2  "THS"
  T_amb/1 -> Subtract2/2  "T_a"
  Gain2/1 -> Sum1/4
  Sum1/1 -> Gain3/1
  Integrator/1 -> [THS]  "THS"
  Subtract4/1 -> Gain5/1
  Subsystem3/2(T_j) -> [T_bl]  "T2_b"
  Sum/1 -> Sum1/1
  Gain4/1 -> Sum2/1
  Subsystem5/1(T_c) -> Subtract6/1  "T4_2"
  [THS] -> Subtract4/2  "THS"
  Subtract5/1 -> Gain6/1
  [THS] -> Subtract3/2  "THS"
  Subtract2/1 -> Gain2/1
  [THS] -> Subtract/2  "THS"
  Gain5/1 -> Sum2/2
  Gain1/1 -> Sum/2
  Subsystem4/2(T_j) -> [T_bh]  "T1_b"
  Sum3/1 -> Sum1/3
  Subsystem3/1(T_c) -> Subtract4/1  "T4_2"
  Subsystem4/1(T_c) -> Subtract3/1  "T4_1"
  Sum2/1 -> Sum1/2
  Gain3/1 -> Integrator/1  "d_THS"
  Subtract3/1 -> Gain4/1
  Subtract1/1 -> Gain1/1
  Subsystem6/2(T_j) -> [T_ch]  "T1_c"
  P_loss/1 -> Selector5/1, Selector4/1, Selector3/1, Selector2/1, Selector1/1, Selector/1
  [T_ah] -> Bus Creator/1  "T_aH"
  [T_ch] -> Bus Creator/5  "T_cH"
  [T_bl] -> Bus Creator/4  "T_bL"
  [T_al] -> Bus Creator/2  "T_aL"
  [T_cl] -> Bus Creator/6  "T_cL"
  Bus Creator/1 -> T_j/1  "T_j"
  [T_bh] -> Bus Creator/3  "T_bH"
  Selector/1 -> Subsystem2/1(P)
  Selector3/1 -> Subsystem3/1(P)
  Selector4/1 -> Subsystem6/1(P)
  Selector5/1 -> Subsystem5/1(P)
  Selector1/1 -> Subsystem1/1(P)
  Selector2/1 -> Subsystem4/1(P)
  [THS] -> Subsystem2/2(THS), Subsystem1/2(THS), Subsystem4/2(THS), Subsystem3/2(THS), Subsystem6/2(THS), Subsystem5/2(THS)  "THS"

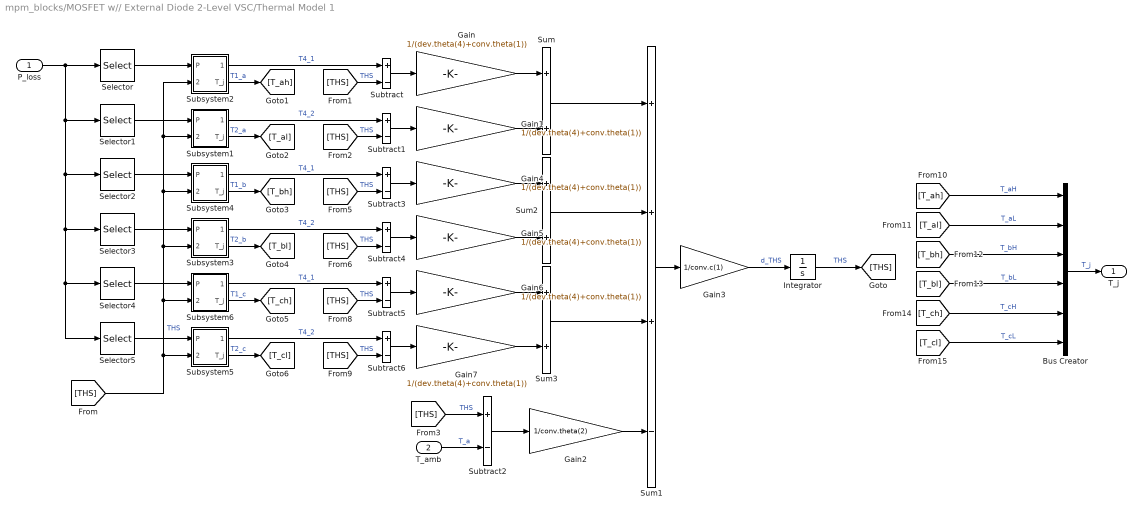
== system mpm_blocks/MOSFET w// External Diode 2-Level VSC/Thermal Model 1 ==
  P_loss : Inport
  T_amb : Inport  Port=2
  Bus Creator : BusCreator  Inputs=6
  Gain{,1,4..7} (6 alike) : Gain  Gain=1/(dev.theta(4)+conv.theta(1))
  Gain2 : Gain  Gain=1/conv.theta(2)
  Gain3 : Gain  Gain=1/conv.c(1)
  Integrator : Integrator  InitialCondition=conv.T_init-273.15
  Selector : Selector  InputPortWidth=6  IndexOptions=Index vector (dialog)  Indices=1  OutputSizes=1
  Selector1 : Selector  InputPortWidth=6  IndexOptions=Index vector (dialog)  Indices=4  OutputSizes=1
  Selector2 : Selector  InputPortWidth=6  IndexOptions=Index vector (dialog)  Indices=2  OutputSizes=1
  Selector3 : Selector  InputPortWidth=6  IndexOptions=Index vector (dialog)  Indices=5  OutputSizes=1
  Selector4 : Selector  InputPortWidth=6  IndexOptions=Index vector (dialog)  Indices=3  OutputSizes=1
  Selector5 : Selector  InputPortWidth=6  IndexOptions=Index vector (dialog)  Indices=6  OutputSizes=1
  Subsystem1 : Subsystem
  Subsystem2 : Subsystem
  Subsystem3 : Subsystem
  Subsystem4 : Subsystem
  Subsystem5 : Subsystem
  Subsystem6 : Subsystem
  Subtract{,1..6} (7 alike) : Sum  Inputs=+-
  Sum : Sum
  Sum1 : Sum  Inputs=+++-
  Sum2 : Sum
  Sum3 : Sum
  T_j : Outport
  wires:
  Subsystem2/1(T_c) -> Subtract/1  "T4_1"
  Subsystem1/1(T_c) -> Subtract1/1  "T4_2"
  Subtract/1 -> Gain/1
  Subsystem2/2(T_j) -> [T_ah]  "T1_a"
  Subsystem6/1(T_c) -> Subtract5/1  "T4_1"
  [THS] -> Subtract5/2  "THS"
  Gain7/1 -> Sum3/2
  Subtract6/1 -> Gain7/1
  Subsystem5/2(T_j) -> [T_cl]  "T2_c"
  [THS] -> Subtract6/2  "THS"
  [THS] -> Subtract2/1  "THS"
  Gain6/1 -> Sum3/1
  Gain/1 -> Sum/1
  Subsystem1/2(T_j) -> [T_al]  "T2_a"
  [THS] -> Subtract1/2  "THS"
  T_amb/1 -> Subtract2/2  "T_a"
  Gain2/1 -> Sum1/4
  Sum1/1 -> Gain3/1
  Integrator/1 -> [THS]  "THS"
  Subtract4/1 -> Gain5/1
  Subsystem3/2(T_j) -> [T_bl]  "T2_b"
  Sum/1 -> Sum1/1
  Gain4/1 -> Sum2/1
  Subsystem5/1(T_c) -> Subtract6/1  "T4_2"
  [THS] -> Subtract4/2  "THS"
  Subtract5/1 -> Gain6/1
  [THS] -> Subtract3/2  "THS"
  Subtract2/1 -> Gain2/1
  [THS] -> Subtract/2  "THS"
  Gain5/1 -> Sum2/2
  Gain1/1 -> Sum/2
  Subsystem4/2(T_j) -> [T_bh]  "T1_b"
  Sum3/1 -> Sum1/3
  Subsystem3/1(T_c) -> Subtract4/1  "T4_2"
  Subsystem4/1(T_c) -> Subtract3/1  "T4_1"
  Sum2/1 -> Sum1/2
  Gain3/1 -> Integrator/1  "d_THS"
  Subtract3/1 -> Gain4/1
  Subtract1/1 -> Gain1/1
  Subsystem6/2(T_j) -> [T_ch]  "T1_c"
  P_loss/1 -> Selector5/1, Selector4/1, Selector3/1, Selector2/1, Selector1/1, Selector/1
  [T_ah] -> Bus Creator/1  "T_aH"
  [T_ch] -> Bus Creator/5  "T_cH"
  [T_bl] -> Bus Creator/4  "T_bL"
  [T_al] -> Bus Creator/2  "T_aL"
  [T_cl] -> Bus Creator/6  "T_cL"
  Bus Creator/1 -> T_j/1  "T_j"
  [T_bh] -> Bus Creator/3  "T_bH"
  Selector/1 -> Subsystem2/1(P)
  Selector3/1 -> Subsystem3/1(P)
  Selector4/1 -> Subsystem6/1(P)
  Selector5/1 -> Subsystem5/1(P)
  Selector1/1 -> Subsystem1/1(P)
  Selector2/1 -> Subsystem4/1(P)
  [THS] -> Subsystem2/2(THS), Subsystem1/2(THS), Subsystem4/2(THS), Subsystem3/2(THS), Subsystem6/2(THS), Subsystem5/2(THS)  "THS"

== system mpm_blocks/MOSFET w// Integrated Diode 2-Level VSC/Calculate Duty & Currents ==
  r_ds : Inport
  v_th : Inport  Port=2
  r_dio : Inport  Port=3
  v_s : Inport  Port=4
  i_s : Inport  Port=5
  v_dc : Inport  Port=6
  Calculate Device Currents : MATLAB Function  TreatAsAtomicUnit=on
  Duty Cycle Estimation : Subsystem
  Gain : Gain  Gain=-1
  Product : Product
  Product1 : Product
  Selector : Selector  InputPortWidth=6  IndexOptions=Index vector (dialog)  Indices=[1 2 3]  OutputSizes=1
  Selector1 : Selector  InputPortWidth=6  IndexOptions=Index vector (dialog)  Indices=[1 2 3]  OutputSizes=1
  Subtract : Sum  Inputs=+-
  Sum of Elements : Sum  Inputs=+
  d_M : Outport
  i_M : Outport  Port=2
  d_D : Outport  Port=3
  i_D : Outport  Port=4
  i_dc : Outport  Port=5
  wires:
  r_dio/1 -> Calculate Device Currents/6(r_dio)
  v_s/1 -> Duty Cycle Estimation/2(v_s)
  Calculate Device Currents/1(i_m) -> i_M/1, Product/2  "i_M"
  Duty Cycle Estimation/2(d_D) -> Calculate Device Currents/2(d_d)  "d_deadTime"
  r_ds/1 -> Calculate Device Currents/4(r_ds)
  v_th/1 -> Calculate Device Currents/5(v_th)
  Duty Cycle Estimation/1(d_M) -> d_M/1, Product/1, Calculate Device Currents/1(d_m)  "d_M"
  i_s/1 -> Calculate Device Currents/3(i_s)
  v_dc/1 -> Duty Cycle Estimation/1(v_dc)
  Calculate Device Currents/3(d_d_new) -> Product1/2, d_D/1  "i_D"
  Calculate Device Currents/2(i_d) -> Product1/1, i_D/1  "d_D"
  Product1/1 -> Selector1/1
  Product/1 -> Selector/1
  Gain/1 -> i_dc/1  "i_dc"
  Sum of Elements/1 -> Gain/1
  Subtract/1 -> Sum of Elements/1  "diff"
  Selector/1 -> Subtract/1
  Selector1/1 -> Subtract/2

== system mpm_blocks/MOSFET w// Integrated Diode 2-Level VSC/DE Loss Modeling ==
  d_D : Inport
  i_D : Inport  Port=2
  r_dio : Inport  Port=3
  v_th : Inport  Port=4
  v_dc : Inport  Port=5
  E_rr : Inport  Port=6
  Gain : Gain  Gain=1/conv.dev(2).V_ref
  Gain3 : Gain  Gain=1/conv.dev(2).I_ref
  Gain4 : Gain  Gain=conv.f_sw
  Product : Product
  Product3 : Product  Inputs=3
  Product6 : Product  Inputs=3
  Product8 : Product
  Sqrt : Sqrt
  Square2 : Math  Operator=square
  Sum : Sum
  Sum2 : Sum
  P_D : Outport
  wires:
  E_rr/1 -> Product3/1
  v_th/1 -> Product8/2
  Sum2/1 -> P_D/1  "P_D"
  Product3/1 -> Gain4/1
  r_dio/1 -> Product6/1
  Gain4/1 -> Sum2/2  "P_SD"
  Sum/1 -> Sum2/1  "P_CD"
  Square2/1 -> Product6/3
  Product8/1 -> Sum/2
  Product6/1 -> Sum/1
  Gain/1 -> Product3/2  "vscale"
  Gain3/1 -> Sqrt/1
  Sqrt/1 -> Product3/3  "iscale"
  d_D/1 -> Product/1, Product6/2  "d_D"
  i_D/1 -> Product/2, Square2/1  "i_D"
  Product/1 -> Product8/1, Gain3/1  "i_D_avg"
  v_dc/1 -> Gain/1

== system mpm_blocks/MOSFET w// Integrated Diode 2-Level VSC/MOSFET Loss Modeling ==
  d_M : Inport
  i_M : Inport  Port=2
  r_ds : Inport  Port=3
  E_sw : Inport  Port=4
  v_dc : Inport  Port=5
  Abs : Abs  SaturateOnIntegerOverflow=off
  Constant : Constant  Value=conv.dev(1).k_v
  Gain : Gain  Gain=1/conv.dev(1).V_ref
  Gain1 : Gain  Gain=conv.f_sw
  Gain2 : Gain  Gain=1/conv.dev(1).I_ref
  Power : Math  Operator=pow
  Product : Product
  Product10 : Product  Inputs=3
  Product4 : Product  Inputs=3
  Square : Math  Operator=square
  Sum1 : Sum
  P_M : Outport
  wires:
  Product4/1 -> Sum1/1  "P_CM"
  Gain2/1 -> Product10/2  "iscale"
  Square/1 -> Product4/3
  Product10/1 -> Gain1/1
  Power/1 -> Product10/3  "vscale"
  r_ds/1 -> Product4/1
  Gain1/1 -> Sum1/2  "P_SM"
  i_M/1 -> Square/1, Product/1  "i_M"
  E_sw/1 -> Product10/1
  Sum1/1 -> P_M/1  "P_M"
  Abs/1 -> Gain2/1
  d_M/1 -> Product/2, Product4/2  "d"
  Product/1 -> Abs/1
  Constant/1 -> Power/2
  Gain/1 -> Power/1
  v_dc/1 -> Gain/1

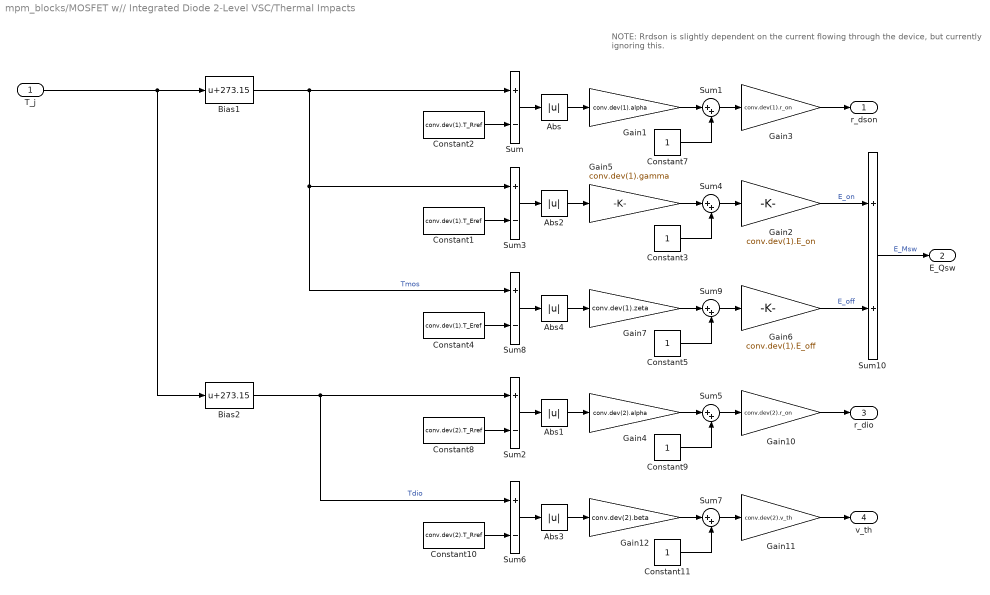
== system mpm_blocks/MOSFET w// Integrated Diode 2-Level VSC/Thermal Impacts ==
  note: NOTE: Rrdson is slightly dependent on the current flowing through the device, but currently ignoring this.
  T_j : Inport
  Abs{,1..4} (5 alike) : Abs  SaturateOnIntegerOverflow=off
  Bias1 : Bias  Bias=273.15  SaturateOnIntegerOverflow=off
  Bias2 : Bias  Bias=273.15  SaturateOnIntegerOverflow=off
  Constant1 : Constant  Value=conv.dev(1).T_Eref
  Constant10 : Constant  Value=conv.dev(2).T_Rref
  Constant{3,5,7,9,11} (5 alike) : Constant
  Constant2 : Constant  Value=conv.dev(1).T_Rref
  Constant4 : Constant  Value=conv.dev(1).T_Eref
  Constant8 : Constant  Value=conv.dev(2).T_Rref
  Gain1 : Gain  Gain=conv.dev(1).alpha
  Gain10 : Gain  Gain=conv.dev(2).r_on
  Gain11 : Gain  Gain=conv.dev(2).v_th
  Gain12 : Gain  Gain=conv.dev(2).beta
  Gain2 : Gain  Gain=conv.dev(1).E_on
  Gain3 : Gain  Gain=conv.dev(1).r_on
  Gain4 : Gain  Gain=conv.dev(2).alpha
  Gain5 : Gain  Gain=conv.dev(1).gamma
  Gain6 : Gain  Gain=conv.dev(1).E_off
  Gain7 : Gain  Gain=conv.dev(1).zeta
  Sum{,2..3,6,8} (5 alike) : Sum  Inputs=+-
  Sum{1,4..5,7,9} (5 alike) : Sum  Inputs=|++
  Sum10 : Sum
  r_dson : Outport
  E_Qsw : Outport  Port=2
  r_dio : Outport  Port=3
  v_th : Outport  Port=4
  wires:
  Sum/1 -> Abs/1
  Gain3/1 -> r_dson/1
  Gain10/1 -> r_dio/1
  Sum5/1 -> Gain10/1
  Abs1/1 -> Gain4/1
  Gain4/1 -> Sum5/1
  Constant9/1 -> Sum5/2
  Constant8/1 -> Sum2/2
  Sum2/1 -> Abs1/1
  Constant7/1 -> Sum1/2
  Sum1/1 -> Gain3/1
  Gain1/1 -> Sum1/1
  Abs/1 -> Gain1/1
  Sum6/1 -> Abs3/1
  Gain12/1 -> Sum7/1
  Constant10/1 -> Sum6/2
  Sum7/1 -> Gain11/1
  Gain11/1 -> v_th/1
  Constant11/1 -> Sum7/2
  Constant2/1 -> Sum/2
  Abs3/1 -> Gain12/1
  Sum3/1 -> Abs2/1
  Constant3/1 -> Sum4/2
  Gain5/1 -> Sum4/1
  Abs2/1 -> Gain5/1
  Gain2/1 -> Sum10/1  "E_on"
  Sum4/1 -> Gain2/1
  Constant1/1 -> Sum3/2
  Constant4/1 -> Sum8/2
  Abs4/1 -> Gain7/1
  Gain6/1 -> Sum10/2  "E_off"
  Sum9/1 -> Gain6/1
  Constant5/1 -> Sum9/2
  Sum8/1 -> Abs4/1
  Gain7/1 -> Sum9/1
  Sum10/1 -> E_Qsw/1  "E_Msw"
  Bias1/1 -> Sum8/1, Sum3/1, Sum/1  "Tmos"
  T_j/1 -> Bias2/1, Bias1/1
  Bias2/1 -> Sum6/1, Sum2/1  "Tdio"

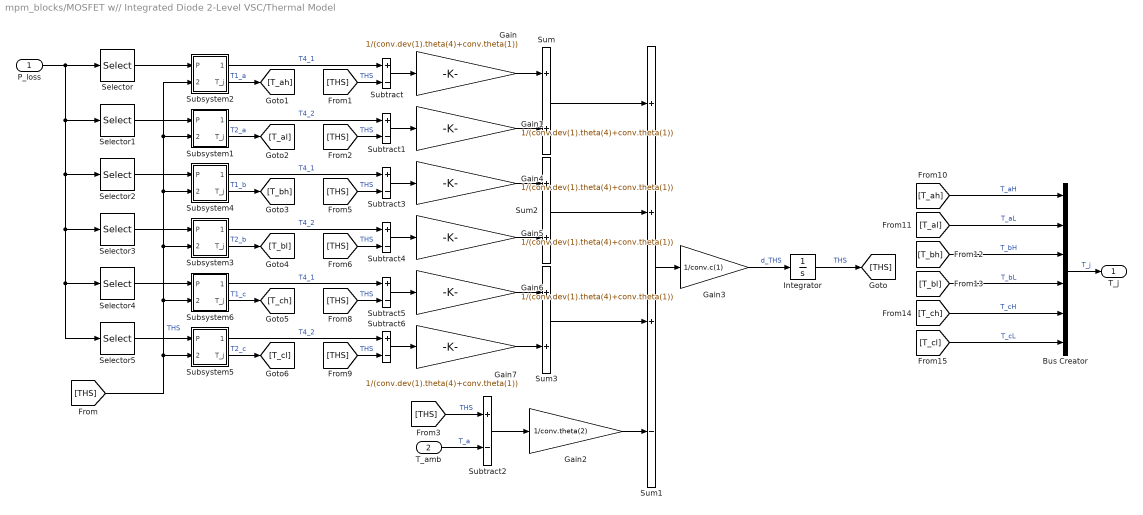
== system mpm_blocks/MOSFET w// Integrated Diode 2-Level VSC/Thermal Model ==
  P_loss : Inport
  T_amb : Inport  Port=2
  Bus Creator : BusCreator  Inputs=6
  Gain{,1,4..7} (6 alike) : Gain  Gain=1/(conv.dev(1).theta(4)+conv.theta(1))
  Gain2 : Gain  Gain=1/conv.theta(2)
  Gain3 : Gain  Gain=1/conv.c(1)
  Integrator : Integrator  InitialCondition=conv.T_init-273.15
  Selector : Selector  InputPortWidth=6  IndexOptions=Index vector (dialog)  Indices=1  OutputSizes=1
  Selector1 : Selector  InputPortWidth=6  IndexOptions=Index vector (dialog)  Indices=4  OutputSizes=1
  Selector2 : Selector  InputPortWidth=6  IndexOptions=Index vector (dialog)  Indices=2  OutputSizes=1
  Selector3 : Selector  InputPortWidth=6  IndexOptions=Index vector (dialog)  Indices=5  OutputSizes=1
  Selector4 : Selector  InputPortWidth=6  IndexOptions=Index vector (dialog)  Indices=3  OutputSizes=1
  Selector5 : Selector  InputPortWidth=6  IndexOptions=Index vector (dialog)  Indices=6  OutputSizes=1
  Subsystem1 : Subsystem
  Subsystem2 : Subsystem
  Subsystem3 : Subsystem
  Subsystem4 : Subsystem
  Subsystem5 : Subsystem
  Subsystem6 : Subsystem
  Subtract{,1..6} (7 alike) : Sum  Inputs=+-
  Sum : Sum
  Sum1 : Sum  Inputs=+++-
  Sum2 : Sum
  Sum3 : Sum
  T_j : Outport
  wires:
  Subsystem2/1(T_c) -> Subtract/1  "T4_1"
  Subsystem1/1(T_c) -> Subtract1/1  "T4_2"
  Subtract/1 -> Gain/1
  Subsystem2/2(T_j) -> [T_ah]  "T1_a"
  Subsystem6/1(T_c) -> Subtract5/1  "T4_1"
  [THS] -> Subtract5/2  "THS"
  Gain7/1 -> Sum3/2
  Subtract6/1 -> Gain7/1
  Subsystem5/2(T_j) -> [T_cl]  "T2_c"
  [THS] -> Subtract6/2  "THS"
  [THS] -> Subtract2/1  "THS"
  Gain6/1 -> Sum3/1
  Gain/1 -> Sum/1
  Subsystem1/2(T_j) -> [T_al]  "T2_a"
  [THS] -> Subtract1/2  "THS"
  T_amb/1 -> Subtract2/2  "T_a"
  Gain2/1 -> Sum1/4
  Sum1/1 -> Gain3/1
  Integrator/1 -> [THS]  "THS"
  Subtract4/1 -> Gain5/1
  Subsystem3/2(T_j) -> [T_bl]  "T2_b"
  Sum/1 -> Sum1/1
  Gain4/1 -> Sum2/1
  Subsystem5/1(T_c) -> Subtract6/1  "T4_2"
  [THS] -> Subtract4/2  "THS"
  Subtract5/1 -> Gain6/1
  [THS] -> Subtract3/2  "THS"
  Subtract2/1 -> Gain2/1
  [THS] -> Subtract/2  "THS"
  Gain5/1 -> Sum2/2
  Gain1/1 -> Sum/2
  Subsystem4/2(T_j) -> [T_bh]  "T1_b"
  Sum3/1 -> Sum1/3
  Subsystem3/1(T_c) -> Subtract4/1  "T4_2"
  Subsystem4/1(T_c) -> Subtract3/1  "T4_1"
  Sum2/1 -> Sum1/2
  Gain3/1 -> Integrator/1  "d_THS"
  Subtract3/1 -> Gain4/1
  Subtract1/1 -> Gain1/1
  Subsystem6/2(T_j) -> [T_ch]  "T1_c"
  P_loss/1 -> Selector5/1, Selector4/1, Selector3/1, Selector2/1, Selector1/1, Selector/1
  [T_ah] -> Bus Creator/1  "T_aH"
  [T_ch] -> Bus Creator/5  "T_cH"
  [T_bl] -> Bus Creator/4  "T_bL"
  [T_al] -> Bus Creator/2  "T_aL"
  [T_cl] -> Bus Creator/6  "T_cL"
  Bus Creator/1 -> T_j/1  "T_j"
  [T_bh] -> Bus Creator/3  "T_bH"
  Selector/1 -> Subsystem2/1(P)
  Selector3/1 -> Subsystem3/1(P)
  Selector4/1 -> Subsystem6/1(P)
  Selector5/1 -> Subsystem5/1(P)
  Selector1/1 -> Subsystem1/1(P)
  Selector2/1 -> Subsystem4/1(P)
  [THS] -> Subsystem2/2(THS), Subsystem1/2(THS), Subsystem4/2(THS), Subsystem3/2(THS), Subsystem6/2(THS), Subsystem5/2(THS)  "THS"
